simulink model "Neurofeedback_Fuzzy_MISO_SemiSyntheticNoise"  (R2022a)
settings: Solver=VariableStepAuto  StartTime=0.0  StopTime=120  MaxStep=1/10  RelTol=1e-3
libraries: dspsrcs4 x4, fuzblock x1
settings Model: Creator=mariodelossantos  LastModifiedBy=mariodelossantos

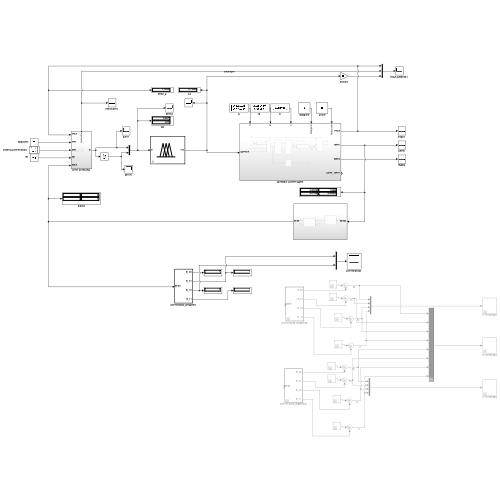
[thumbnail: Simulink's stored preview of the top-level diagram]
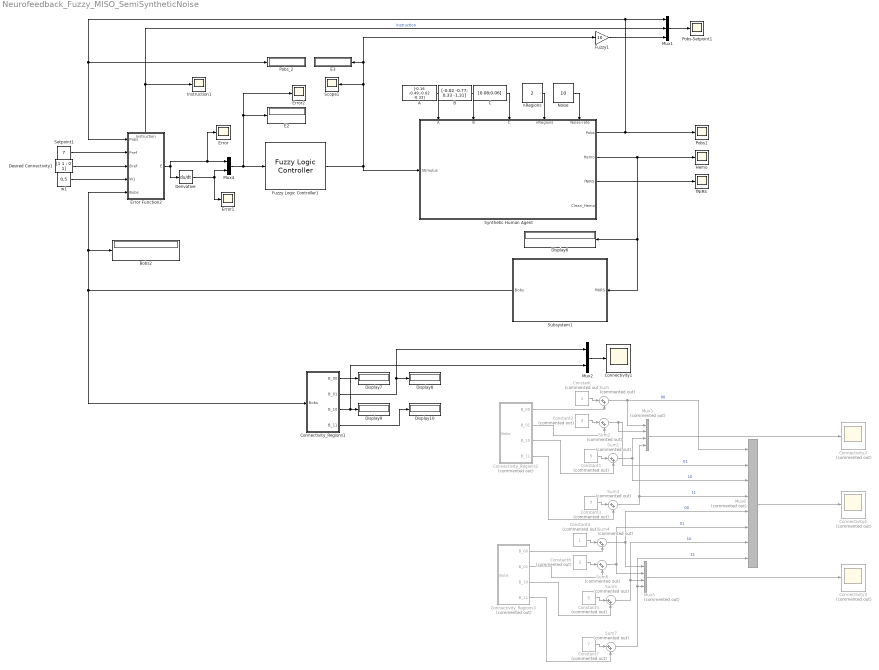
== system Neurofeedback_Fuzzy_MISO_SemiSyntheticNoise ==
  A : Constant  Value=[-0.16 -0.49;-0.02 -0.33]
  B : Constant  Value=[-0.02 -0.77; 0.33 -1.31]
  Bobs2 : Display
  C : Constant  Value=[0.08;0.06]
  Connectivity1 : Scope
  Connectivity2 : Scope  Commented=on
  Connectivity3 : Scope  Commented=on
  Connectivity4 : Scope  Commented=on
  Connectivity_Regions1 : MATLAB Function  TreatAsAtomicUnit=on
  Connectivity_Regions2 : MATLAB Function  Commented=on  TreatAsAtomicUnit=on
  Connectivity_Regions3 : MATLAB Function  Commented=on  TreatAsAtomicUnit=on
  Constant : Constant  Commented=on
  Constant1 : Constant  Commented=on  Value=5
  Constant2 : Constant  Commented=on  Value=3
  Constant3 : Constant  Commented=on  Value=7
  Constant4 : Constant  Commented=on
  Constant5 : Constant  Commented=on  Value=5
  Constant6 : Constant  Commented=on  Value=3
  Constant7 : Constant  Commented=on  Value=7
  Derivative : Derivative  CoefficientInTFapproximation=1
  Desired Connectivity1 : Constant  Value="[1   1 ; 0  1]"
  Display{6..10} (5 alike) : Display
  E2 : Display
  E3 : Display
  Error : Scope
  Error Function2 : Subsystem
      settings: PortSchema="{\"entries\":[{\"content\":{\"sides\":[{\"content\":{\"connectorIds\":[\"In1\",\"In2\",\"In3\",\"In4\",\"In5\"]},\"type\":\"ConnectorPlacement.EquallySpacedRectSide\",\"uuid\":\"444fbf9f-83f0-405e-b780-73f2a519e5d8\"},{\"content\":{\"connectorIds\":[\"Out1\"],\"side\":\"RIGHT\"},\"type\":\"ConnectorPlacement.EquallySpacedRectSide\",\"uuid\":\"580feeb9-eb76-4e38-ada2-7c0fba9b3602\"},{\"content\":{\"connectorIds\":[\"Out2\"],\"side\":\"TOP\"},\"type\":\"ConnectorPlacement.EquallySpacedRectSide\",\"uuid\":\"86f5bef5-f023-4b75-b93f-dc016b73225e\"}]},\"type\":\"ConnectorPlacement.EquallySpacedConnector\",\"uuid\":\"50bb9fda-b7f3-427b-ab4c-df885dc392aa\"}],\"packageUris\":[\"http://schema.mathworks.com/mf0/Connector/R2020b\"],\"version\":\"1.0\"}"
  Error1 : Scope
  Error2 : Scope
  Fuzzy Logic Controller1 : fuzblock/Fuzzy Logic  Controller  FIS=cFNIRS_MISO_v4  OutputSampleNumber=101  DataType=double  FuzzifiedInputs=off  RuleFiringStrengths=off  RuleOutputs=off  AggregatedOutputs=off  SimulateUsing=Interpreted execution  OutOfRangeInputValueMessage=warning  NoRuleFiredMessage=warning  EmptyOutputFuzzySetMessage=warning
  Fuzzy1 : Gain  Gain=10
  Hemo : Scope
  Instruction1 : Scope
  Mux1 : Mux  Inputs=3
  Mux2 : Mux  Inputs=2
  Mux3 : Mux  Commented=on
  Mux4 : Mux  Inputs=2
  Mux5 : Mux  Commented=on
  Mux6 : Mux  Commented=on  Inputs=8
  Noise : Constant  Value=10
  Pobs-Setpoint1 : Scope
  Pobs1 : Scope
  Pobs_2 : Display
  Scope1 : Scope
  Setpoint1 : Constant  Value=7
  Subsystem1 : Subsystem
  Sum{,1..7} (8 alike) : Sum  Commented=on  Inputs=|++
  Synthetic Human Agent : Subsystem
      settings: PortSchema="{\"entries\":[{\"content\":{\"sides\":[{\"content\":{\"connectorIds\":[\"In1\"]},\"type\":\"ConnectorPlacement.EquallySpacedRectSide\",\"uuid\":\"bfbcc5e8-6241-430f-b542-d1842988c81e\"},{\"content\":{\"connectorIds\":[\"Out1\",\"Out2\",\"Out3\",\"Out4\"],\"side\":\"RIGHT\"},\"type\":\"ConnectorPlacement.EquallySpacedRectSide\",\"uuid\":\"5787ae13-1686-4c0f-bd71-92bd424cb6c3\"},{\"content\":{\"connectorIds\":[\"In2\",\"In3\",\"In4\",\"In5\",\"In6\"],\"side\":\"TOP\"},\"type\":\"ConnectorPlacement.EquallySpacedRectSide\",\"uuid\":\"d1dd531e-b262-408a-a912-471f5b03e825\"}]},\"type\":\"ConnectorPlacement.EquallySpacedConnector\",\"uuid\":\"b2c21004-90c2-4258-a219-9564d29dafe7\"}],\"packageUris\":[\"http://schema.mathworks.com/mf0/Connector/R2020b\"],\"version\":\"1.0\"}"
  fNIRS : Scope
  nRegions : Constant  Value=2
  w1 : Constant  Value=0.5
  wires:
  Error Function2/1(E) -> Error/1, Mux4/1, Derivative/1
  Mux1/1 -> Pobs-Setpoint1/1
  Connectivity_Regions1/1(B_00) -> Display7/1
  Error Function2/2(Instruction) -> Instruction1/1, Mux1/2  "Instruction"
  C/1 -> Synthetic Human Agent/4(C)
  Desired Connectivity1/1 -> Error Function2/3(Bref)
  Connectivity_Regions1/3(B_10) -> Mux2/2, Display9/1
  A/1 -> Synthetic Human Agent/2(A)
  B/1 -> Synthetic Human Agent/3(B)
  Fuzzy1/1 -> Mux1/3
  Synthetic Human Agent/3(fNIRS) -> fNIRS/1
  Setpoint1/1 -> Error Function2/2(Pref)
  Synthetic Human Agent/1(Pobs) -> Pobs1/1, Error Function2/1(Pobs), Pobs_2/1, Mux1/1
  Fuzzy Logic Controller1/1 -> E3/1, Fuzzy1/1, Scope1/1, Synthetic Human Agent/1(Stimulus)
  Mux2/1 -> Connectivity1/1
  Synthetic Human Agent/2(Hemo) -> Subsystem1/1(fNIRS), Display6/1, Hemo/1
  Subsystem1/1(Bobs) -> Error Function2/5(Bobs), Bobs2/1, Connectivity_Regions1/1(Bobs)
  Connectivity_Regions1/4(B_11) -> Display10/1
  Connectivity_Regions1/2(B_01) -> Mux2/1, Display8/1
  w1/1 -> Error Function2/4(W1)
  Mux4/1 -> Error2/1, E2/1, Fuzzy Logic Controller1/1
  Derivative/1 -> Mux4/2, Error1/1
  Noise/1 -> Synthetic Human Agent/6(Noise-rate)
  nRegions/1 -> Synthetic Human Agent/5(nRegions)
  Mux3/1 -> Connectivity2/1
  Constant/1 -> Sum/1
  Constant1/1 -> Sum1/1
  Constant2/1 -> Sum2/1
  Constant3/1 -> Sum3/1
  Sum/1 -> Mux6/1, Mux3/1  "00"
  Sum2/1 -> Mux6/2, Mux3/2  "01"
  Sum1/1 -> Mux3/3, Mux6/3  "10"
  Sum3/1 -> Mux6/4, Mux3/4  "11"
  Connectivity_Regions2/1(B_00) -> Sum/2
  Connectivity_Regions2/2(B_01) -> Sum2/2
  Connectivity_Regions2/3(B_10) -> Sum1/2
  Connectivity_Regions2/4(B_11) -> Sum3/2
  Mux5/1 -> Connectivity3/1
  Sum4/1 -> Mux6/5, Mux5/1  "00"
  Constant5/1 -> Sum5/1
  Constant7/1 -> Sum7/1
  Constant4/1 -> Sum4/1
  Sum5/1 -> Mux6/7, Mux5/3  "10"
  Connectivity_Regions3/3(B_10) -> Sum5/2
  Connectivity_Regions3/4(B_11) -> Sum7/2
  Sum7/1 -> Mux6/8, Mux5/4  "11"
  Connectivity_Regions3/2(B_01) -> Sum6/2
  Constant6/1 -> Sum6/1
  Connectivity_Regions3/1(B_00) -> Sum4/2
  Sum6/1 -> Mux5/2, Mux6/6  "01"
  Mux6/1 -> Connectivity4/1

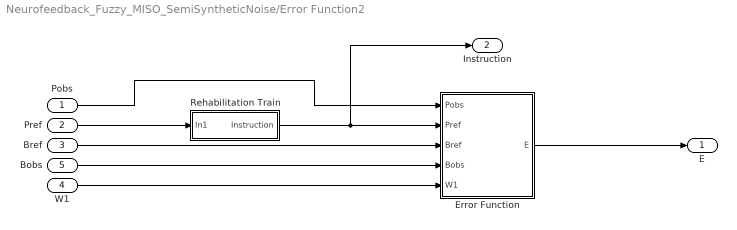
== system Neurofeedback_Fuzzy_MISO_SemiSyntheticNoise/Error Function2 ==
  Pobs : Inport
  Pref : Inport  Port=2
  Bref : Inport  Port=3
  W1 : Inport  Port=4
  Bobs : Inport  Port=5
  Error Function : Subsystem
  Rehabilitation Train : Subsystem
  E : Outport
  Instruction : Outport  Port=2
  wires:
  Bobs/1 -> Error Function/4(Bobs)
  W1/1 -> Error Function/5(W1)
  Pref/1 -> Rehabilitation Train/1(In1)
  Pobs/1 -> Error Function/1(Pobs)
  Rehabilitation Train/1(Instruction) -> Instruction/1, Error Function/2(Pref)
  Error Function/1(E) -> E/1
  Bref/1 -> Error Function/3(Bref)

== system Neurofeedback_Fuzzy_MISO_SemiSyntheticNoise/Subsystem1 ==
  fNIRS : Inport
  DQ1 : Scope
  Incremental_Avg_Boot1 : Subsystem
  Threshold : Constant  Value=0.6
  getConnectivity_Validation1 : MATLAB Function  TreatAsAtomicUnit=on  SystemSampleTime=0
  Bobs : Outport
  wires:
  getConnectivity_Validation1/1(Bobs) -> Bobs/1
  fNIRS/1 -> Incremental_Avg_Boot1/1(fNIRS)
  Incremental_Avg_Boot1/1("D ") -> getConnectivity_Validation1/1("D ")
  getConnectivity_Validation1/2(DQ) -> DQ1/1
  Threshold/1 -> getConnectivity_Validation1/2(Threshold)

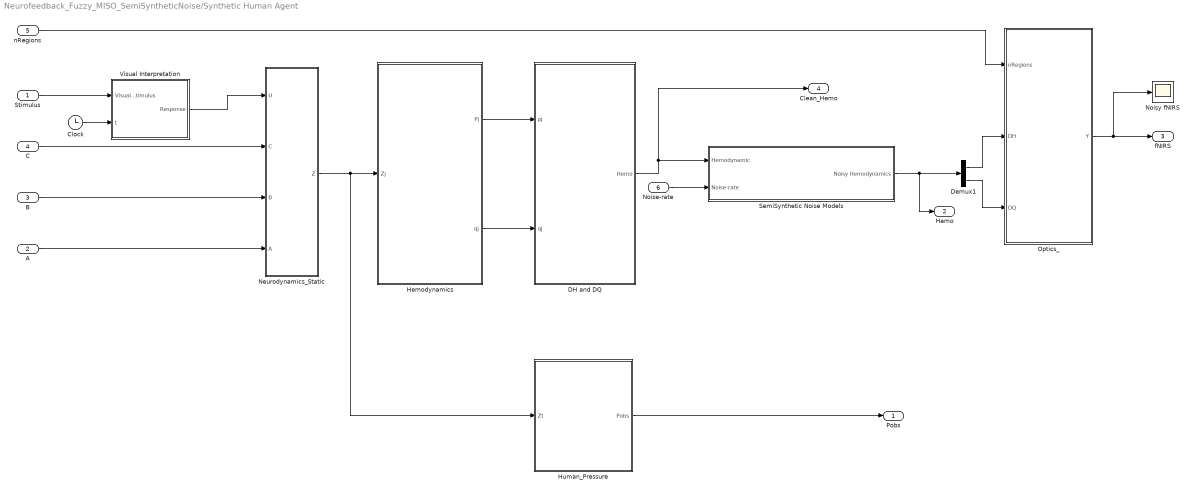
== system Neurofeedback_Fuzzy_MISO_SemiSyntheticNoise/Synthetic Human Agent ==
  Stimulus : Inport
  A : Inport  Port=2
  B : Inport  Port=3
  C : Inport  Port=4
  nRegions : Inport  Port=5
  Noise-rate : Inport  Port=6
  Clock : Clock
  DH and DQ : Subsystem
  Demux1 : Demux  Outputs=2
  Hemodynamics : Subsystem
  Human_Pressure : Subsystem
  Neurodynamics_Static : Subsystem
  Noisy fNIRS : Scope
  Optics_ : MATLAB Function  TreatAsAtomicUnit=on
  SemiSynthetic Noise Models : Subsystem
  Visual Interpretation : MATLAB Function  TreatAsAtomicUnit=on
  Pobs : Outport
  Hemo : Outport  Port=2
  fNIRS : Outport  Port=3
  Clean_Hemo : Outport  Port=4
  wires:
  DH and DQ/1(Hemo) -> SemiSynthetic Noise Models/1(Hemodynamic), Clean_Hemo/1
  Hemodynamics/1(Pj) -> DH and DQ/1(pj)
  nRegions/1 -> Optics_/1(nRegions)
  C/1 -> Neurodynamics_Static/2(C)
  Hemodynamics/2(qj) -> DH and DQ/2(qj)
  A/1 -> Neurodynamics_Static/4(A)
  Human_Pressure/1(Pobs) -> Pobs/1
  B/1 -> Neurodynamics_Static/3(B)
  Neurodynamics_Static/1(Z) -> Human_Pressure/1(Zt), Hemodynamics/1(Zj)
  Demux1/1 -> Optics_/2(DH)
  Demux1/2 -> Optics_/3(DQ)
  Optics_/1(Y) -> Noisy fNIRS/1, fNIRS/1
  SemiSynthetic Noise Models/1(Noisy Hemodynamics) -> Demux1/1, Hemo/1
  Noise-rate/1 -> SemiSynthetic Noise Models/2(Noise-rate)
  Clock/1 -> Visual Interpretation/2(t)
  Stimulus/1 -> Visual Interpretation/1(Visual_Stimulus)
  Visual Interpretation/1(Response) -> Neurodynamics_Static/1(U)

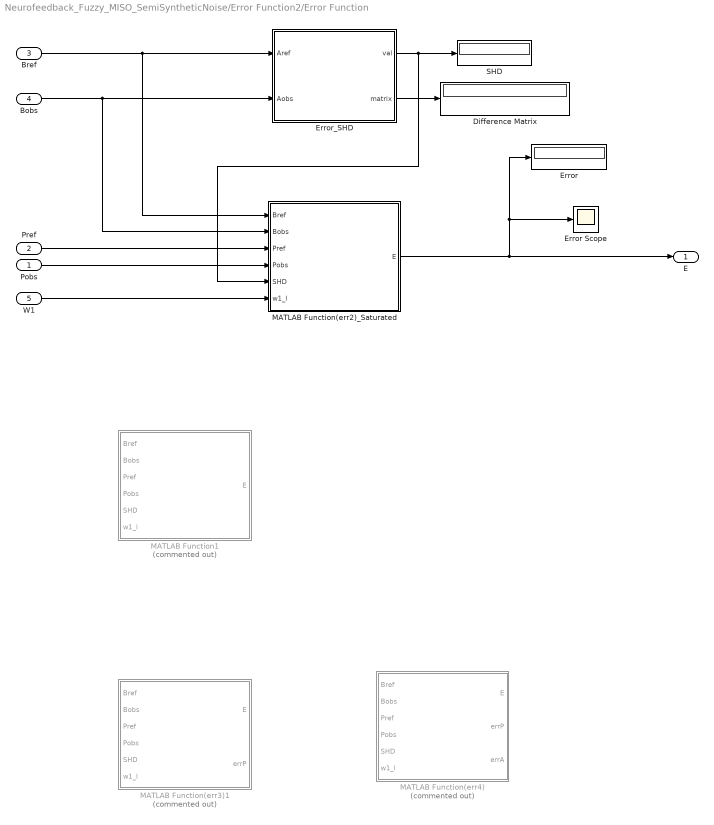
== system Neurofeedback_Fuzzy_MISO_SemiSyntheticNoise/Error Function2/Error Function ==
  Pobs : Inport
  Pref : Inport  Port=2
  Bref : Inport  Port=3
  Bobs : Inport  Port=4
  W1 : Inport  Port=5
  Difference Matrix : Display
  Error : Display
  Error Scope : Scope
  Error_SHD : MATLAB Function  TreatAsAtomicUnit=on
  MATLAB Function(err2)_Saturated : MATLAB Function  TreatAsAtomicUnit=on
  MATLAB Function(err3)1 : MATLAB Function  Commented=on  TreatAsAtomicUnit=on
  MATLAB Function(err4) : MATLAB Function  Commented=on  TreatAsAtomicUnit=on
  MATLAB Function1 : MATLAB Function  Commented=on  TreatAsAtomicUnit=on
  SHD : Display
  E : Outport
  wires:
  Error_SHD/2(matrix) -> Difference Matrix/1
  Bref/1 -> MATLAB Function(err2)_Saturated/1(Bref), Error_SHD/1(Aref)
  Error_SHD/1(val) -> MATLAB Function(err2)_Saturated/5(SHD), SHD/1
  Bobs/1 -> MATLAB Function(err2)_Saturated/2(Bobs), Error_SHD/2(Aobs)
  Pobs/1 -> MATLAB Function(err2)_Saturated/4(Pobs)
  Pref/1 -> MATLAB Function(err2)_Saturated/3(Pref)
  W1/1 -> MATLAB Function(err2)_Saturated/6(w1_l)
  MATLAB Function(err2)_Saturated/1(E) -> Error/1, Error Scope/1, E/1

== system Neurofeedback_Fuzzy_MISO_SemiSyntheticNoise/Error Function2/Rehabilitation Train ==
  In1 : Inport
  Duty_Cycle_U1 : Constant  Value=0.166667  OutMin=[0]  OutMax=[0.8]
  Period_Time_U1 : Constant  Value=30
  Setpoint_follow : Product
  Variable Pulse Generator2 : VariablePulseGenerator  AllowZeroPulseWidth=on  RunAtFixedTimeIntervals=on  SampleTime=1/10
  Instruction : Outport
  wires:
  Duty_Cycle_U1/1 -> Variable Pulse Generator2/1
  In1/1 -> Setpoint_follow/2
  Period_Time_U1/1 -> Variable Pulse Generator2/2
  Setpoint_follow/1 -> Instruction/1
  Variable Pulse Generator2/1 -> Setpoint_follow/1

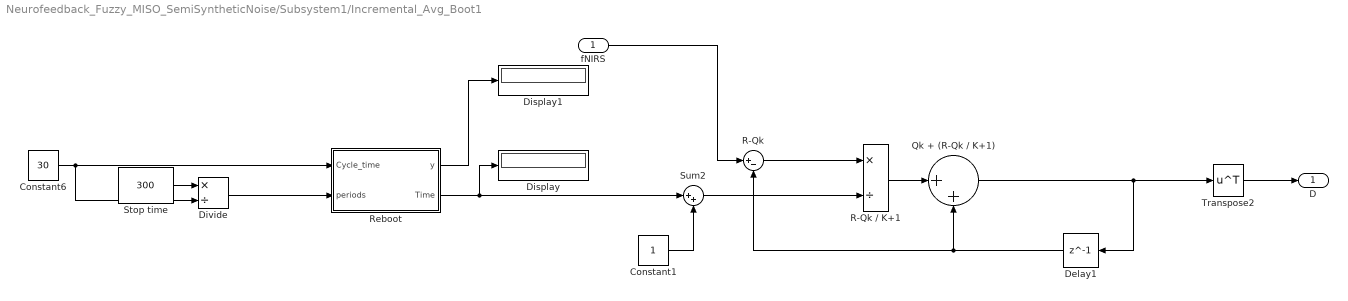
== system Neurofeedback_Fuzzy_MISO_SemiSyntheticNoise/Subsystem1/Incremental_Avg_Boot1 ==
  fNIRS : Inport
  Constant1 : Constant
  Constant6 : Constant  Value=30
  Delay1 : Delay  DelayLength=1  InitialCondition=[0 0 0 0]
  Display : Display
  Display1 : Display
  Divide : Product  Inputs=*/
  "Qk + (R-Qk / K+1) " : Sum  Inputs=|++
  R-Qk : Sum  Inputs=|+-
  R-Qk / K+1 : Product  Inputs=*/
  Reboot : Subsystem
  Stop time : Constant  Value=300
  Sum2 : Sum  Inputs=|++
  Transpose2 : Math  Operator=transpose
  "D " : Outport
  wires:
  Constant1/1 -> Sum2/2
  fNIRS/1 -> R-Qk/1
  R-Qk / K+1/1 -> "Qk + (R-Qk / K+1) "/1
  Sum2/1 -> R-Qk / K+1/2
  R-Qk/1 -> R-Qk / K+1/1
  Delay1/1 -> R-Qk/2, "Qk + (R-Qk / K+1) "/2
  Reboot/2(Time) -> Sum2/1, Display/1
  Constant6/1 -> Reboot/1(Cycle_time), Divide/2
  Reboot/1(y) -> Display1/1
  Divide/1 -> Reboot/2(periods)
  Stop time/1 -> Divide/1
  Transpose2/1 -> "D "/1
  "Qk + (R-Qk / K+1) "/1 -> Delay1/1, Transpose2/1

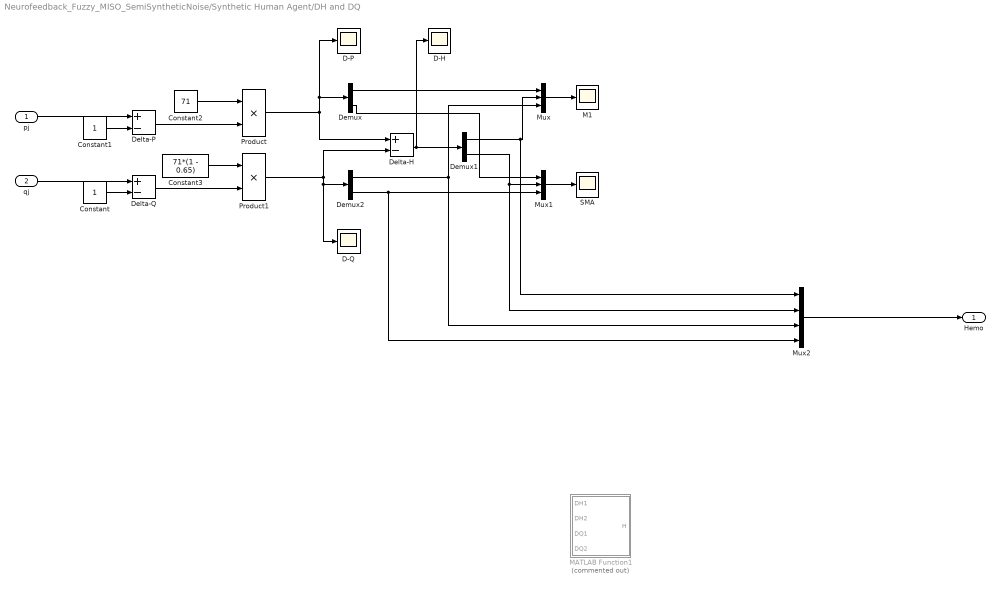
== system Neurofeedback_Fuzzy_MISO_SemiSyntheticNoise/Synthetic Human Agent/DH and DQ ==
  pj : Inport
  qj : Inport  Port=2
  Constant : Constant
  Constant1 : Constant
  Constant2 : Constant  Value=71
  Constant3 : Constant  Value=71*(1 - 0.65)
  D-H : Scope
  D-P : Scope
  D-Q : Scope
  Delta-H : Sum  Inputs=+-
  Delta-P : Sum  Inputs=+-
  Delta-Q : Sum  Inputs=+-
  Demux : Demux  Outputs=2
  Demux1 : Demux  Outputs=2
  Demux2 : Demux  Outputs=2
  M1 : Scope
  MATLAB Function1 : MATLAB Function  Commented=on  TreatAsAtomicUnit=on
  Mux : Mux  Inputs=3
  Mux1 : Mux  Inputs=3
  Mux2 : Mux
  Product : Product
  Product1 : Product
  SMA : Scope
  Hemo : Outport
  wires:
  Constant2/1 -> Product/1
  Delta-Q/1 -> Product1/2
  Constant3/1 -> Product1/1
  Demux2/2 -> Mux2/4, Mux1/3
  pj/1 -> Delta-P/1
  Mux1/1 -> SMA/1
  Demux/2 -> Mux1/1
  Mux/1 -> M1/1
  Constant/1 -> Delta-Q/2
  Delta-P/1 -> Product/2
  Product1/1 -> Demux2/1, D-Q/1, Delta-H/2
  qj/1 -> Delta-Q/1
  Demux/1 -> Mux/1
  Delta-H/1 -> Demux1/1, D-H/1
  Demux1/1 -> Mux2/1, Mux/2
  Demux1/2 -> Mux2/2, Mux1/2
  Product/1 -> Demux/1, D-P/1, Delta-H/1
  Demux2/1 -> Mux2/3, Mux/3
  Constant1/1 -> Delta-P/2
  Mux2/1 -> Hemo/1

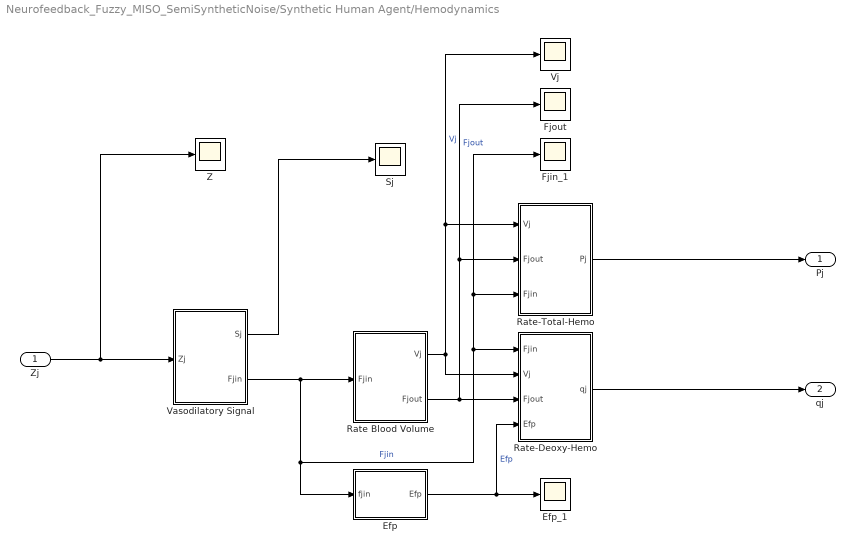
== system Neurofeedback_Fuzzy_MISO_SemiSyntheticNoise/Synthetic Human Agent/Hemodynamics ==
  Zj : Inport
  Efp : MATLAB Function  TreatAsAtomicUnit=on
  Efp_1 : Scope
  Fjin_1 : Scope
  Fjout : Scope
  Rate Blood Volume : Subsystem
  Rate-Deoxy-Hemo : Subsystem
  Rate-Total-Hemo : Subsystem
  Sj : Scope
  Vasodilatory Signal : Subsystem
  Vj : Scope
  Z : Scope
  Pj : Outport
  qj : Outport  Port=2
  wires:
  Rate-Deoxy-Hemo/1(qj) -> qj/1
  Zj/1 -> Vasodilatory Signal/1(Zj), Z/1
  Vasodilatory Signal/1(Sj) -> Sj/1
  Rate Blood Volume/2(Fjout) -> Fjout/1, Rate-Total-Hemo/2(Fjout), Rate-Deoxy-Hemo/3(Fjout)  "Fjout"
  Rate Blood Volume/1(Vj) -> Vj/1, Rate-Total-Hemo/1(Vj), Rate-Deoxy-Hemo/2(Vj)  "Vj"
  Rate-Total-Hemo/1(Pj) -> Pj/1
  Efp/1(Efp) -> Rate-Deoxy-Hemo/4(Efp), Efp_1/1  "Efp"
  Vasodilatory Signal/2(Fjin) -> Efp/1(fjin), Fjin_1/1, Rate-Total-Hemo/3(Fjin), Rate-Deoxy-Hemo/1(Fjin), Rate Blood Volume/1(Fjin)  "Fjin"

== system Neurofeedback_Fuzzy_MISO_SemiSyntheticNoise/Synthetic Human Agent/Human_Pressure ==
  Zt : Inport
  Clock : Clock
  Gain : Gain  Gain=10
  Pressure Generator : MATLAB Function  TreatAsAtomicUnit=on
  SENSOR : MATLAB Function  TreatAsAtomicUnit=on
  Scope : Scope
  Scope1 : Scope
  Pobs : Outport
  wires:
  Clock/1 -> Pressure Generator/2(t)
  Zt/1 -> Pressure Generator/1(Zt)
  SENSOR/1(Pobs) -> Scope1/1, Gain/1
  Pressure Generator/1(Pobs) -> SENSOR/1(Vout), Scope/1
  Gain/1 -> Pobs/1

== system Neurofeedback_Fuzzy_MISO_SemiSyntheticNoise/Synthetic Human Agent/Neurodynamics_Static ==
  U : Inport
  C : Inport  Port=2
  B : Inport  Port=3
  A : Inport  Port=4
  Integrator : Integrator
  Jt : MATLAB Function  TreatAsAtomicUnit=on
  Product1 : Product  Multiplication=Matrix(*)
  Sum : Sum  Inputs=|++
  Z : Outport
  wires:
  Integrator/1 -> Jt/1(Zt), Z/1
  Product1/1 -> Sum/1
  Jt/1(Jt) -> Sum/2
  Sum/1 -> Integrator/1
  U/1 -> Jt/2(U), Product1/2
  C/1 -> Product1/1
  A/1 -> Jt/4(A_input)
  B/1 -> Jt/3(B_input)

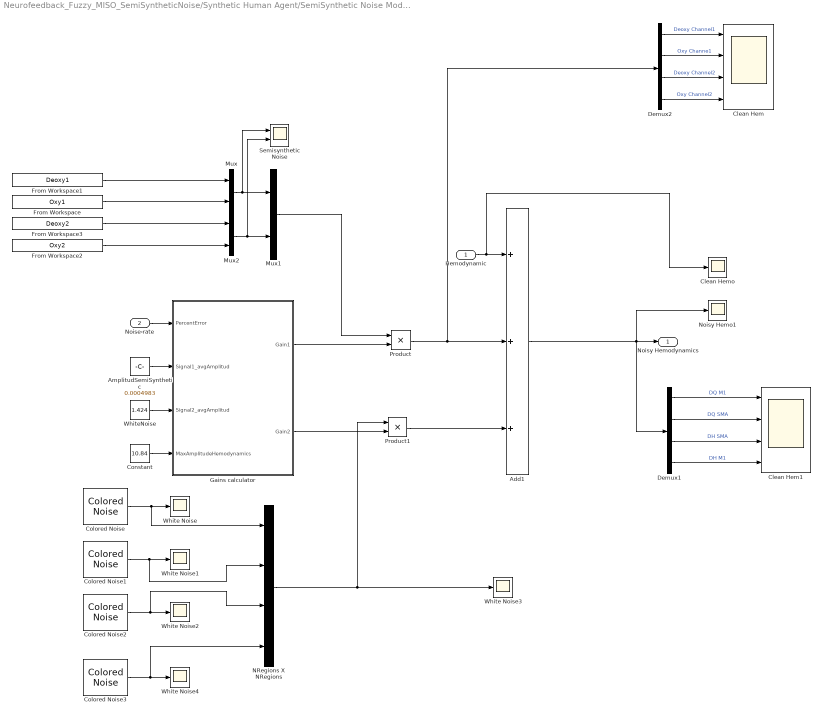
== system Neurofeedback_Fuzzy_MISO_SemiSyntheticNoise/Synthetic Human Agent/SemiSynthetic Noise Models ==
  Hemodynamic : Inport
  Noise-rate : Inport  Port=2
  Add1 : Sum  Inputs=+++
  AmplitudSemiSynthetic : Constant  Value=0.0004983
  Clean Hem : Scope  NumInputPorts=4
  Clean Hem1 : Scope  NumInputPorts=4
  Clean Hemo : Scope
  Colored Noise : dspsrcs4/Colored Noise  Color=white  InverseFrequencyPower=1  BoundedOutput=on  NumChannels=1  OutputDataType=double  SamplesPerFrame=1  SampleTime=1/10  RandomStream=mt19937ar with seed  Seed=67  SimulateUsing=Interpreted execution
      settings: SourceProductBaseCode=DS
  Colored Noise1 : dspsrcs4/Colored Noise  Color=white  InverseFrequencyPower=1  BoundedOutput=on  NumChannels=1  OutputDataType=double  SamplesPerFrame=1  SampleTime=1/10  RandomStream=mt19937ar with seed  Seed=40  SimulateUsing=Interpreted execution
      settings: SourceProductBaseCode=DS
  Colored Noise2 : dspsrcs4/Colored Noise  Color=white  InverseFrequencyPower=1  BoundedOutput=on  NumChannels=1  OutputDataType=double  SamplesPerFrame=1  SampleTime=1/10  RandomStream=mt19937ar with seed  Seed=41  SimulateUsing=Interpreted execution
      settings: SourceProductBaseCode=DS
  Colored Noise3 : dspsrcs4/Colored Noise  Color=white  InverseFrequencyPower=1  BoundedOutput=on  NumChannels=1  OutputDataType=double  SamplesPerFrame=1  SampleTime=1/10  RandomStream=mt19937ar with seed  Seed=50  SimulateUsing=Interpreted execution
      settings: SourceProductBaseCode=DS
  Constant : Constant  Value=10.84
  Demux1 : Demux
  Demux2 : Demux
  From Workspace : FromWorkspace  VariableName=Oxy1  OutputAfterFinalValue=Holding final value
  From Workspace1 : FromWorkspace  VariableName=Deoxy1
  From Workspace2 : FromWorkspace  VariableName=Oxy2  OutputAfterFinalValue=Holding final value
  From Workspace3 : FromWorkspace  VariableName=Deoxy2
  Gains calculator : MATLAB Function  TreatAsAtomicUnit=on
  Mux : Mux  Inputs=2
  Mux1 : Mux  Inputs=2
  Mux2 : Mux  Inputs=2
  NRegions X NRegions : Mux
  Noisy Hemo1 : Scope
  Product : Product
  Product1 : Product
  Semisynthetic Noise : Scope  NumInputPorts=2
  White Noise{,1..4} (5 alike) : Scope
  WhiteNoise : Constant  Value=1.424
  Noisy Hemodynamics : Outport
  wires:
  Gains calculator/1(Gain1) -> Product/2
  Noise-rate/1 -> Gains calculator/1(PercentError)
  Add1/1 -> Demux1/1, Noisy Hemodynamics/1, Noisy Hemo1/1
  AmplitudSemiSynthetic/1 -> Gains calculator/2(Signal1_avgAmplitud)
  Hemodynamic/1 -> Clean Hemo/1, Add1/1
  Constant/1 -> Gains calculator/4(MaxAmplitudeHemodynamics)
  Colored Noise/1 -> NRegions X NRegions/1, White Noise/1
  Colored Noise1/1 -> NRegions X NRegions/2, White Noise1/1
  Colored Noise2/1 -> NRegions X NRegions/3, White Noise2/1
  NRegions X NRegions/1 -> Product1/1, White Noise3/1
  Colored Noise3/1 -> NRegions X NRegions/4, White Noise4/1
  Gains calculator/2(Gain2) -> Product1/2
  WhiteNoise/1 -> Gains calculator/3(Signal2_avgAmplitud)
  From Workspace/1 -> Mux/2
  Product1/1 -> Add1/3
  Mux/1 -> Mux1/1, Semisynthetic Noise/1
  From Workspace1/1 -> Mux/1
  From Workspace3/1 -> Mux2/1
  From Workspace2/1 -> Mux2/2
  Mux2/1 -> Mux1/2, Semisynthetic Noise/2
  Mux1/1 -> Product/1
  Demux2/3 -> Clean Hem/3  "Deoxy Channel2"
  Product/1 -> Add1/2, Demux2/1
  Demux2/2 -> Clean Hem/2  "Oxy Channe1"
  Demux2/4 -> Clean Hem/4  "Oxy Channel2"
  Demux2/1 -> Clean Hem/1  "Deoxy Channel1"
  Demux1/1 -> Clean Hem1/1  "DQ M1"
  Demux1/2 -> Clean Hem1/2  "DQ SMA"
  Demux1/3 -> Clean Hem1/3  "DH SMA"
  Demux1/4 -> Clean Hem1/4  "DH M1"

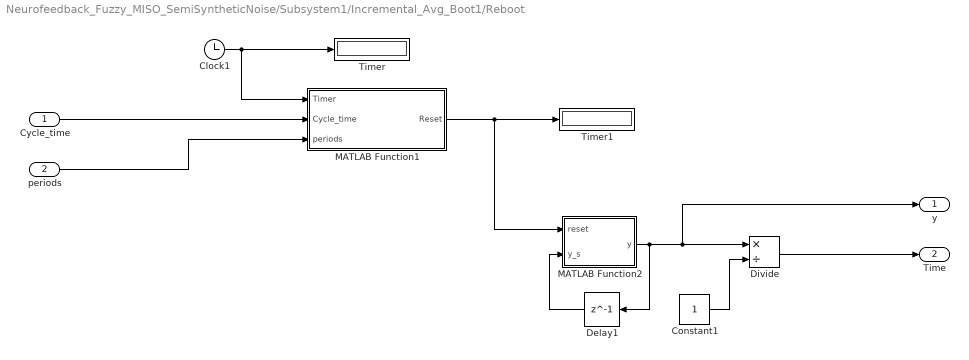
== system Neurofeedback_Fuzzy_MISO_SemiSyntheticNoise/Subsystem1/Incremental_Avg_Boot1/Reboot ==
  Cycle_time : Inport
  periods : Inport  Port=2
  Clock1 : Clock
  Constant1 : Constant
  Delay1 : Delay  DelayLength=1
  Divide : Product  Inputs=*/
  MATLAB Function1 : MATLAB Function  TreatAsAtomicUnit=on
  MATLAB Function2 : MATLAB Function  TreatAsAtomicUnit=on
  Timer : Display
  Timer1 : Display
  y : Outport
  Time : Outport  Port=2
  wires:
  MATLAB Function1/1(Reset) -> MATLAB Function2/1(reset), Timer1/1
  MATLAB Function2/1(y) -> y/1, Divide/1, Delay1/1
  Constant1/1 -> Divide/2
  Clock1/1 -> MATLAB Function1/1(Timer), Timer/1
  periods/1 -> MATLAB Function1/3(periods)
  Delay1/1 -> MATLAB Function2/2(y_s)
  Divide/1 -> Time/1
  Cycle_time/1 -> MATLAB Function1/2(Cycle_time)

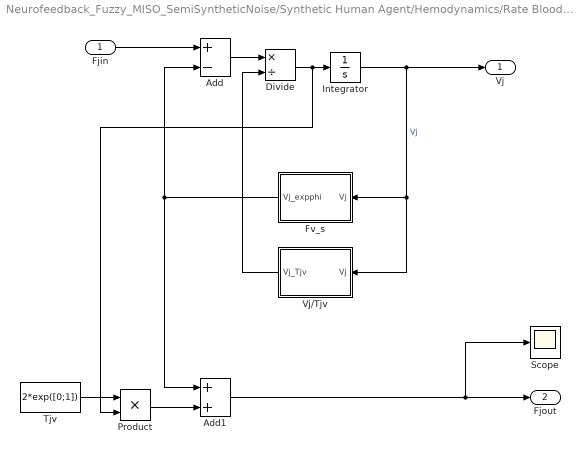
== system Neurofeedback_Fuzzy_MISO_SemiSyntheticNoise/Synthetic Human Agent/Hemodynamics/Rate Blood Volume ==
  Fjin : Inport
  Add : Sum  Inputs=+-
  Add1 : Sum
  Divide : Product  Inputs=*/
  Fv_s : MATLAB Function  TreatAsAtomicUnit=on
  Integrator : Integrator  InitialCondition=exp([0;0])
  Product : Product
  Scope : Scope
  Tjv : Constant  Value=2*exp([0;1])
  Vj/Tjv : MATLAB Function  TreatAsAtomicUnit=on
  Vj : Outport
  Fjout : Outport  Port=2
  wires:
  Fjin/1 -> Add/1
  Integrator/1 -> Vj/1, Vj/Tjv/1(Vj), Fv_s/1(Vj)  "Vj"
  Divide/1 -> Product/2, Integrator/1
  Fv_s/1(Vj_expphi) -> Add/2, Add1/1
  Add/1 -> Divide/1
  Vj/Tjv/1(Vj_Tjv) -> Divide/2
  Product/1 -> Add1/2
  Tjv/1 -> Product/1
  Add1/1 -> Scope/1, Fjout/1

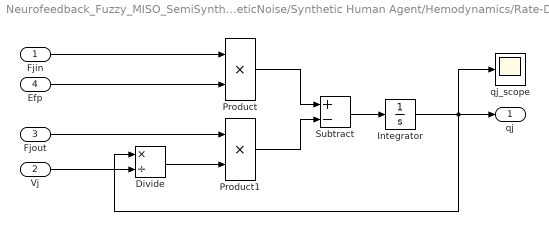
== system Neurofeedback_Fuzzy_MISO_SemiSyntheticNoise/Synthetic Human Agent/Hemodynamics/Rate-Deoxy-Hemo ==
  Fjin : Inport
  Vj : Inport  Port=2
  Fjout : Inport  Port=3
  Efp : Inport  Port=4
  Divide : Product  Inputs=*/
  Integrator : Integrator  InitialCondition=exp([0;0])
  Product : Product
  Product1 : Product
  Subtract : Sum  Inputs=+-
  qj_scope : Scope
  qj : Outport
  wires:
  Efp/1 -> Product/2
  Divide/1 -> Product1/2
  Subtract/1 -> Integrator/1
  Integrator/1 -> qj/1, Divide/1, qj_scope/1
  Vj/1 -> Divide/2
  Product1/1 -> Subtract/2
  Fjin/1 -> Product/1
  Fjout/1 -> Product1/1
  Product/1 -> Subtract/1

== system Neurofeedback_Fuzzy_MISO_SemiSyntheticNoise/Synthetic Human Agent/Hemodynamics/Rate-Total-Hemo ==
  Vj : Inport
  Fjout : Inport  Port=2
  Fjin : Inport  Port=3
  Divide : Product  Inputs=*/
  Integrator : Integrator  InitialCondition=exp([0;0])
  Product : Product
  Subtract : Sum  Inputs=+-
  pj : Scope
  Pj : Outport
  wires:
  Fjout/1 -> Subtract/2
  Product/1 -> Integrator/1
  Vj/1 -> Divide/2
  Subtract/1 -> Product/1
  Fjin/1 -> Subtract/1
  Divide/1 -> Product/2
  Integrator/1 -> Pj/1, pj/1, Divide/1

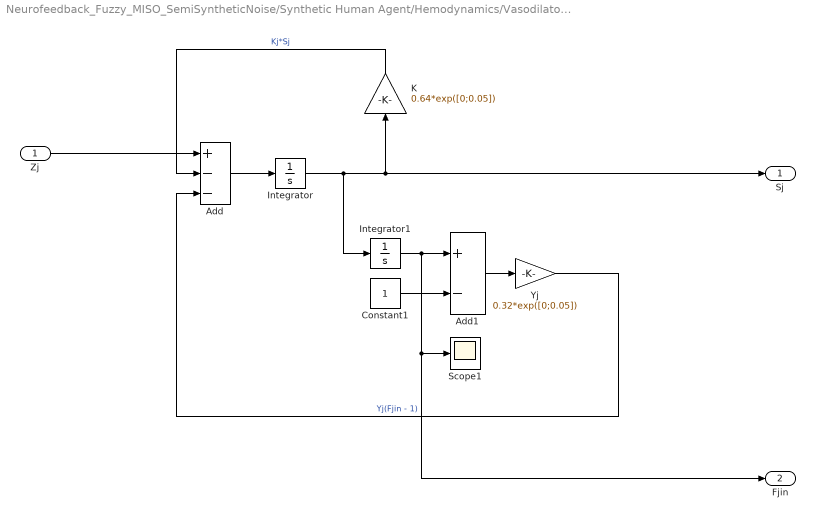
== system Neurofeedback_Fuzzy_MISO_SemiSyntheticNoise/Synthetic Human Agent/Hemodynamics/Vasodilatory Signal ==
  Zj : Inport
  Add : Sum  Inputs=+--
  Add1 : Sum  Inputs=+-
  Constant1 : Constant
  Integrator : Integrator
  Integrator1 : Integrator  InitialCondition=exp([0;0])
  K : Gain  Gain=0.64*exp([0;0.05])
  Scope1 : Scope
  Yj : Gain  Gain=0.32*exp([0;0.05])
  Sj : Outport
  Fjin : Outport  Port=2
  wires:
  Add1/1 -> Yj/1
  K/1 -> Add/2  "Kj*Sj"
  Constant1/1 -> Add1/2
  Zj/1 -> Add/1
  Integrator1/1 -> Fjin/1, Scope1/1, Add1/1
  Integrator/1 -> Sj/1, K/1, Integrator1/1
  Add/1 -> Integrator/1
  Yj/1 -> Add/3  "Yj(Fjin - 1)"

== matlab function Neurofeedback_Fuzzy_MISO_SemiSyntheticNoise/Synthetic Human Agent/Visual Interpretation ==
  data: Visual_Stimulus input; Response output; t input
function Response = fcn(Visual_Stimulus, t)
    R=17.5; %Resistor [Ohms] 10k 
    C= 0.65; %Capacitor [Faradays] 1mF
    V= Visual_Stimulus; %Voltage or system reference;
    Vc = V * (1- exp(-t/(R*C))); % Voltage at the capacitor  
    
Response = Vc;

== matlab function Neurofeedback_Fuzzy_MISO_SemiSyntheticNoise/Subsystem1/Incremental_Avg_Boot1/Reboot/MATLAB Function1 ==
  data: Timer input; Reset output; Cycle_time input; periods input
function Reset  = fcn(Timer, Cycle_time, periods)

temp = 0;
PCycles = zeros(periods,1);
for i = 1:periods
    PCycles(i) = i * Cycle_time;
    if (Timer >= PCycles(i) && Timer <= PCycles(i)+1)
        temp = 1;
        break
    else
        temp = 0;
    end
end 
Reset = temp;

== matlab function Neurofeedback_Fuzzy_MISO_SemiSyntheticNoise/Connectivity_Regions2 ==
  data: Bobs input; B_00 output; B_01 output; B_10 output; B_11 output
function [B_00, B_01, B_10, B_11] = fcn(Bobs)


B_00 = (Bobs(1,1));
B_01 = (Bobs(1,2));
B_10 = (Bobs(2,1));
B_11 = (Bobs(2,2));

== matlab function Neurofeedback_Fuzzy_MISO_SemiSyntheticNoise/Synthetic Human Agent/Hemodynamics/Efp ==
  data: fjin input; Efp output
function Efp= fcn(fjin)

Efp = (1 - (1 - 0.32).^ (1 ./ fjin))/0.32;

== matlab function Neurofeedback_Fuzzy_MISO_SemiSyntheticNoise/Subsystem1/Incremental_Avg_Boot1/Reboot/MATLAB Function2 ==
  data: reset input; y_s input; y output
function y = fcn(reset, y_s)

if reset == 1
    y = 0;
else 
    y = (y_s + 1);
end

== matlab function Neurofeedback_Fuzzy_MISO_SemiSyntheticNoise/Subsystem1/getConnectivity_Validation1 ==
  data: D input; Bobs output; DQ output; Threshold input
function [Bobs,DQ]  = getConnectivity(D, Threshold)

    DQ = zeros(1, 2);
    DQ(1,1)=D(1,1);
    DQ(1,2)=D(1,2);


    DH = zeros(1,2);
    DH(1,1)=D(1,3);
    DH(1,2)=D(1,4);

    rThresh= Threshold; % [0..1] A threshold on the correlation.

    [~,nChannels, nHb]=size(DQ);

    C = nan(nChannels, nChannels, nHb); %Matrix of channel pairwise correlations;

    %This part of the algorithm is HIGHLY inefficient but it does the job for now
    %but might not be sufficiently fast for "real time" neurofeedback

    for iHb = 1:nHb
        for iCh=1:nChannels
            for jCh=iCh:nChannels

                if iCh == jCh

                 C(iCh,jCh,iHb) = 1;

                else

                 C(iCh,jCh,iHb) = xcorr2(DQ(:,iCh,iHb),DQ(:,jCh,iHb));

                end
            end

        end

    end

    %Threshold/Binarize C


    tmp = C > rThresh;

    %Finally "merge" accross Hb species

    Bobs = all(tmp,3); %Apply the AND function across Hb species.

== matlab function Neurofeedback_Fuzzy_MISO_SemiSyntheticNoise/Connectivity_Regions3 ==
  data: Bobs input; B_00 output; B_01 output; B_10 output; B_11 output
function [B_00, B_01, B_10, B_11] = fcn(Bobs)


B_00 = (Bobs(1,1));
B_01 = (Bobs(1,2));
B_10 = (Bobs(2,1));
B_11 = (Bobs(2,2));

== matlab function Neurofeedback_Fuzzy_MISO_SemiSyntheticNoise/Synthetic Human Agent/Hemodynamics/Rate Blood Volume/Fv_s ==
  data: Vj input; Vj_expphi output
function Vj_expphi = fcn(Vj)
phi = 0.32;
Vj_expphi = Vj.^(1/phi);

== matlab function Neurofeedback_Fuzzy_MISO_SemiSyntheticNoise/Synthetic Human Agent/Hemodynamics/Rate Blood Volume/Vj//Tjv ==
  data: Vj input; Vj_Tjv output
function Vj_Tjv = fcn(Vj)
    Tjv = 2*exp([0;1]);
    Tj = 2*exp([0;0.05]);
Vj_Tjv =(Tj.*Tjv.*Vj);

== matlab function Neurofeedback_Fuzzy_MISO_SemiSyntheticNoise/Synthetic Human Agent/Human_Pressure/Pressure Generator ==
  data: Zt input; Pobs output; t input
function Pobs = fcn(Zt, t)
    R=10000; %Resistor [Ohms];
    C= 2; %Capacitor [Faradays];
    V= Zt(1); %Voltage or system reference;
    Vc = V * (exp(-t/(R*C))); % Voltage at the capacitor  
    
Pobs = Vc;

== matlab function Neurofeedback_Fuzzy_MISO_SemiSyntheticNoise/Error Function2/Error Function/MATLAB Function(err3)1 ==
  data: Bref input; E output size=1; Bobs input; Pref input; Pobs input; SHD input; w1_l input; errP output
function [E, errP]  = ErrorFunction(Bref, Bobs, Pref, Pobs, SHD, w1_l)
    w1 = w1_l; %Use whatever values you like most. Threshold 

    w2 = 1 - w1;

    assert(all(size(Bref) == size(Bobs)));

    assert(size(Bref,1) == size(Bref,2));

    nChannels = size(Bref,1);

    BfullyConnected = ones(nChannels);

    BfullyDisconnected = zeros(nChannels);

   
    maxDiffSHD= sum(sum(xor(BfullyConnected,BfullyDisconnected))); %SHD
    errA = SHD/maxDiffSHD; %Normalize error in the connectivity
    %errP = (abs(Pref-Pobs))/abs(Pref);

    %errP = exp(-1/(Pobs - Pref) + eps);

    errP = -(Pref-Pobs) * exp(-(Pref-Pobs)^2);
    
    
    
E = w1 * errA + abs(w2 * errP);

== matlab function Neurofeedback_Fuzzy_MISO_SemiSyntheticNoise/Synthetic Human Agent/Human_Pressure/SENSOR ==
  data: Vout input; Pobs output
function Pobs  = PressureGenerator_sensor(Vout)

    Vcc = 50; %Considering 5V as a real sensor, the value is on mV
    Rf = 100; %Fixed resistor 10k ohms
    kgf = 0.1019716213; % 1N = 0.1019716213 kgf
    Fsr = 0;
    Fsrforce = 0;
    Fsr = (Vcc - Vout * Rf) / Vout;
    FsConductance = 1000000; %Sensor conductance in uOhms
    FsConductance = FsConductance / Fsr;
    if FsConductance <= 1000
        Fsrforce = FsConductance / 80; %Force on Newtons
    else
        Fsrforce = FsConductance - 1000;
        Fsrforce = Fsrforce / 30;
    end
    
Pobs = Fsrforce * kgf;

end

== matlab function Neurofeedback_Fuzzy_MISO_SemiSyntheticNoise/Synthetic Human Agent/Neurodynamics_Static/Jt ==
  data: Zt input; U input; Jt output; B_input input; A_input input
function Jt = fcn(Zt, U, B_input, A_input)
   A = A_input;
   nRegions  = size(A,1);
   M = size(U,1); %nStimuli
   simulationLength = size(U,2);
   %NOTE: Consider that in case of have more than one stimulus, you must
   %change this. 
   B = B_input;
   T = zeros(nRegions); %nRegions x nRegions
    for t = 1:simulationLength
           for uu = 1:M % Sum (Uj * Bj)
               tmp = U(uu,t)*B(:,:,uu);
               T = -0.5*exp(T + tmp);  
           end
    end
    SI = diag(A);
    A =  A - diag(exp(SI) + SI);
Jt = ((A + T)*Zt);

== matlab function Neurofeedback_Fuzzy_MISO_SemiSyntheticNoise/Synthetic Human Agent/Optics_ ==
  data: nRegions input; DH input; DQ input; Y output
function Y  = Optical_Changes(nRegions,DH, DQ)
%% Version V1
% Authors - Mario De Los Santos, Felipe Orihuela-Espina, Javier Herrara-Vega
% Date - March, 2022
% Email - madlsh3517@gmail.com
% Based on: 2015 Stak DCM for fNIRS.
%
%% Input Parameters
% DQ - HbR - Rate of deoxy-hemoglobin
% DH - HbT - Total Hemoglobin
%
%% Output Parameters
% y- optical density changes 
%
%% 

%Using simulink is not possible to have a dynamic matrix that we can
%iterate based on the nRegions variable, but you could easly replace the
%number of regions in the variable "Regions" according your needs
Regions = 2;
Y = zeros(Regions,Regions);
tempDHQ = zeros(nRegions, 2);


% We are using as L1 = 780nm and as L2 = 850nm (same as STak for the
% second one)
%Based on: Giannoni, L., Lange, F., & Tachtsidis, I. (2020). Investigation of the quantification 
% of hemoglobin and cytochrome-c-oxidase in the exposed cortex with near-infrared hyperspectral imaging: 
% a simulation study. Journal of biomedical optics, 25(4), 046001.

F_P =[(0.0007358251*7.5) (0.001104715*6.5) ; (0.001159306*7.5) (0.0007858993*6.5)]; 

%Itereation between regions, nRegions is given as constant by the user.
for i = 1:nRegions
    tempDHQ(:,i) = DQ(i);
    tempDHQ(:,i) = DH(i);
    Y(:,:) = F_P * tempDHQ;
end

== matlab function Neurofeedback_Fuzzy_MISO_SemiSyntheticNoise/Error Function2/Error Function/MATLAB Function(err4) ==
  data: Bref input; E output size=1; Bobs input; Pref input; Pobs input; SHD input; w1_l input; errP output; errA output
function [E, errP, errA]  = ErrorFunction(Bref, Bobs, Pref, Pobs, SHD, w1_l)
    w1 = w1_l; %Use whatever values you like most. Threshold 

    w2 = 1 - w1;

    assert(all(size(Bref) == size(Bobs)));

    assert(size(Bref,1) == size(Bref,2));

    nChannels = size(Bref,1);

    BfullyConnected = ones(nChannels);

    BfullyDisconnected = zeros(nChannels);

   
    maxDiffSHD= sum(sum(xor(BfullyConnected,BfullyDisconnected))); %SHD

    errA = SHD/maxDiffSHD; %Normalize error in the connectivity
    %errP = (abs(Pref-Pobs))/abs(Pref);

    %errP = exp(-1/(Pobs - Pref) + eps);

    errP = ((Pref) .* exp(-(Pref).^2)) - (-(Pobs) .* exp(-(Pobs).^2));
    
    
    
E = w1 * errA + w2 * errP;

== matlab function Neurofeedback_Fuzzy_MISO_SemiSyntheticNoise/Error Function2/Error Function/MATLAB Function(err2)_Saturated ==
  data: Bref input; E output size=1; Bobs input; Pref input; Pobs input; SHD input; w1_l input
function E  = ErrorFunction(Bref, Bobs, Pref, Pobs, SHD, w1_l)
    w1 = w1_l; %Use whatever values you like most. Threshold 

    w2 = 1 - w1;

    assert(all(size(Bref) == size(Bobs)));

    assert(size(Bref,1) == size(Bref,2));

    nChannels = size(Bref,1);

    BfullyConnected = ones(nChannels);

    BfullyDisconnected = zeros(nChannels);

   
    maxDiffSHD= sum(sum(xor(BfullyConnected,BfullyDisconnected))); %SHD
    errA = SHD/maxDiffSHD; %Normalize error in the connectivity
    %errP = (abs(Pref-Pobs))/abs(Pref);

    %errP = exp(-1/(Pobs - Pref) + eps);
    %tmp = Pref;
    errP = 0;
    if Pref == 0
        Pref = 0.0005;
    else
        errP = exp (1 / abs(Pref-Pobs)/abs(Pref));
      if errP > 1
            errP = 1;
      end
    end
    %errP = (abs(Pref-Pobs))/abs(tmp);
    
    
E = (w1 * errA + w2 * errP);

== matlab function Neurofeedback_Fuzzy_MISO_SemiSyntheticNoise/Connectivity_Regions1 ==
  data: Bobs input; B_00 output; B_01 output; B_10 output; B_11 output
function [B_00, B_01, B_10, B_11] = fcn(Bobs)


B_00 = (Bobs(1,1));
B_01 = (Bobs(1,2));
B_10 = (Bobs(2,1));
B_11 = (Bobs(2,2));

== matlab function Neurofeedback_Fuzzy_MISO_SemiSyntheticNoise/Synthetic Human Agent/DH and DQ/MATLAB Function1 ==
  data: DH1 input; H output; DH2 input; DQ1 input; DQ2 input
function H = hemo(DH1, DH2, DQ1, DQ2)
H = zeros(1,4);

H(1,1) = DQ1;
H(1,2) = DQ2;
H(1,3) = DH1;
H(1,4) = DH2;

== matlab function Neurofeedback_Fuzzy_MISO_SemiSyntheticNoise/Error Function2/Error Function/Error_SHD ==
  data: Aref input; val output; Aobs input; matrix output
function [val,matrix]=SHD(Aref,Aobs)

val = sum(sum(xor(Aref,Aobs)));
matrix = xor(Aref,Aobs);

== matlab function Neurofeedback_Fuzzy_MISO_SemiSyntheticNoise/Synthetic Human Agent/SemiSynthetic Noise Models/Gains calculator ==
  settings: updateMethod=DISCRETE
  data: PercentError input; Signal1_avgAmplitud input; Signal2_avgAmplitud input; Gain1 output; MaxAmplitudeHemodynamics input; Gain2 output
function [Gain1, Gain2] = Noise_gains(PercentError, Signal1_avgAmplitud, Signal2_avgAmplitud, MaxAmplitudeHemodynamics)

Gain1 = ((MaxAmplitudeHemodynamics / 100) * PercentError)/ Signal1_avgAmplitud;

Gain2 = ((MaxAmplitudeHemodynamics /100)* PercentError) / Signal2_avgAmplitud;

== matlab function Neurofeedback_Fuzzy_MISO_SemiSyntheticNoise/Error Function2/Error Function/MATLAB Function1 ==
  data: Bref input; E output size=1; Bobs input; Pref input; Pobs input; SHD input; w1_l input
function E  = ErrorFunction(Bref, Bobs, Pref, Pobs, SHD, w1_l)
    w1 = w1_l; %Use whatever values you like most. Threshold 

    w2 = 1 - w1;

    assert(all(size(Bref) == size(Bobs)));

    assert(size(Bref,1) == size(Bref,2));

    nChannels = size(Bref,1);

    BfullyConnected = ones(nChannels);

    BfullyDisconnected = zeros(nChannels);

   
    maxDiffSHD= sum(sum(xor(BfullyConnected,BfullyDisconnected))); %SHD
    errA = SHD/maxDiffSHD; %Normalize error in the connectivity

    %errP = abs(Pref-Pobs)/(Pref);

    errP = abs(exp(-1/((Pref-Pobs)) + eps));
    %errP = erf(Pref-Pobs)/erf(Pref);
    
E = (w1 * errA + w2 * errP);
